simulink model "power_HEMS"  (R2017b)
settings: Solver=ode23tb  StartTime=0.0  StopTime=6  RelTol=1e-3  EnableMultiTasking=on
PreLoadFcn:
  | % Data of Solar Panel
  | %5000[W]/130[W]
  | % Total power generated by solar panel reaches 5[KW].
  | % each solar panel generates power 130[kW].
  | V = [0    40 80 120 160 180 200 217 240 260 280];
  | I = 5000/130*[0.68 0.675 0.67 0.665 0.660 0.655 0.640 0.6 0.48 0.28 0];
  | 
  | %subplot(211);plot(V,I);xlabel('Voltage[V]');ylabel('Current[a]')
  | %subplot(212);plot(V.*I);title('Power[W]')
  | 
  | % Sample Time[s]
  | Ts =5e-6;
  | 
  | 
  | %MPPT + PV Control
  | % PI control pamameter of Voltage control(Outer loop)
  | Kp_V = 50e-3;
  | Ki_V = 10;
  | 
  | % PI Control pamameter of Current control(Inner loop)
  | Kp_I = 25e-3;
  | Ki_I = 10;
  | 
  | % Utility Interconnection Control
  | % PI Control pamameter of Voltage control(Outer loop)
  | Kp_V2 = 0.01;
  | Ki_V2 = 25;
  | 
  | % PI control pamameter of Current control(Inner loop)
  | Kp_I2 = 0.01;
  | Ki_I2 = 25;
  | 
  | 
  | % Difference of voltege using in MPPT
  | dV = 0.5;
  | 
  | % Battery Control
  | % PI Control pamameter of Voltage control(Outer loop)
  | Kp_VB = 0.4;
  | Ki_VB = 2;
  | 
  | % PI control pamameter of Current control(Inner loop)
  | Kp_IB = 0.1;
  | Ki_IB = 0.5;
undefined symbols (not defined in the file or in its folder): Angle, Ion, Lithium, Magnitude, sigbuilder_block
libraries: powerlib x47, powerlib_meascontrol x8, simulink x6, electricdrivelib x1, simulink_extras x1
Description:
  | Copyright 2008-2017 The MathWorks, Inc.
settings Model: SimulationMode=accelerator  Creator=MathWorks  LastModifiedBy=solan
settings SolverCC: ZeroCrossControl=DisableAll  ZeroCrossAlgorithm=Adaptive
settings DataIOCC: LimitDataPoints=on  SaveFormat=Array  SignalLoggingSaveFormat=ModelDataLogs
settings OptimizationCC: ExpressionDepthLimit=2147483647  LifeSpan=inf
settings DebuggingCC: UnderspecifiedInitializationDetection=Classic  MergeDetectMultiDrivingBlocksExec=none  SolverPrmCheckMsg=warning  FcnCallInpInsideContextMsg=warning  AllowSymbolicDim=off  StateNameClashWarn=warning  SFUnexpectedBacktrackingDiag=warning  SFNoUnconditionalDefaultTransitionDiag=warning  SFExecutionAtInitializationDiag=none
settings HardwareCC: ProdBitPerPointer=32  ProdBitPerSizeT=32  ProdBitPerPtrDiffT=32  ProdLargestAtomicFloat=None  ProdIntDivRoundTo=Undefined  ProdEndianess=Unspecified  ProdWordSize=32  ProdHWDeviceType=32-bit Generic
settings ModelReferenceCC: PropagateSignalLabelsOutOfModel=off
settings SFSimCC: SimParseCustomCode=off
settings CodeAppCC: StateflowObjectComments=on
settings GRTTargetCC: TargetLangStandard=C89/C90 (ANSI)  GeneratePreprocessorConditionals=Disable all  CombineOutputUpdateFcns=off  GRTInterface=on
settings ConfigComp: CovMetricSettings=dw  CovHtmlReporting=on  CovSaveCumulativeToWorkspaceVar=on  CovSaveSingleToWorkspaceVar=on  CovShowResultsExplorer=off  CovExternalEMLEnable=off  CovSFcnEnable=off
settings SimscapeCC: SimscapeNormalizeSystem=off

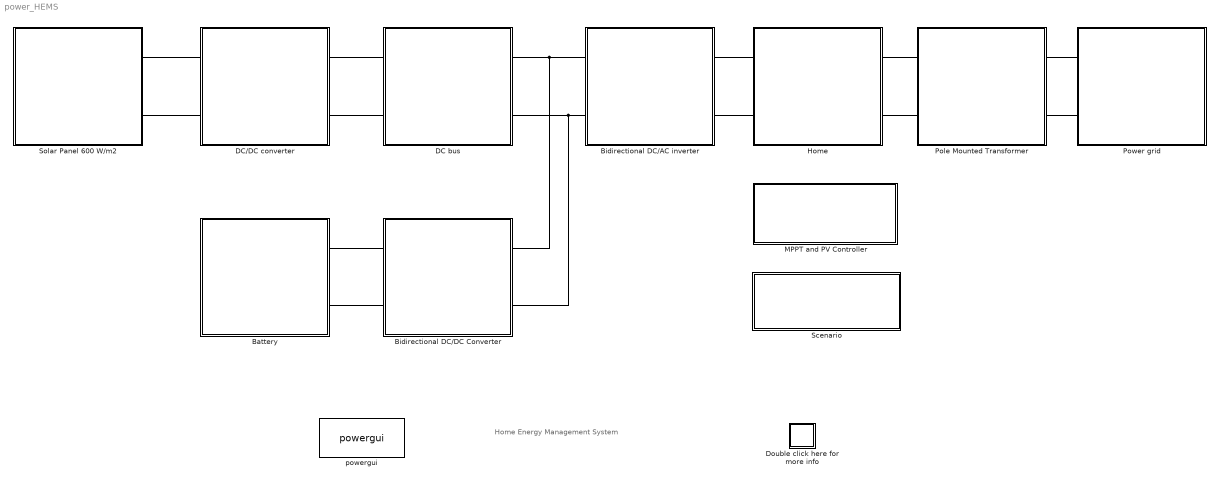
== system power_HEMS ==
  note: Home Energy Management System
  Battery : Subsystem
      mask Display: image(imread('Battery.jpg'))
  Bidirectional DC/AC inverter : Subsystem
      mask Display: image(imread('dcac.jpg'))
  Bidirectional DC/DC Converter : Subsystem
      mask Display: image(imread('bdcdc.jpg'))
  DC bus : Subsystem
      mask Display: image(imread('HVDC.jpg'))
  DC/DC converter : Subsystem
      mask Display: image(imread('dcdc.jpg'))
  Double click here for more info : Subsystem
      settings: OpenFcn=showdemo(bdroot(gcb))
      mask Display: disp('?')
  Home : Subsystem
      mask Display: image(imread('house.jpg'))
  MPPT and PV Controller : Subsystem
      mask Display: disp('Management system')
  Pole Mounted Transformer : Subsystem
      mask Display: image(imread('trans.jpg'))
  Power grid : Subsystem
      mask Display: image(imread('powersystem.jpg'))
  Scenario : Subsystem
      mask Display: disp('Additional\nScopes')
  Solar Panel 600 W/m2 : Subsystem
      mask Display: image(imread('pv.jpg'))
  powergui : powerlib/powergui  Priority=1  SimulationMode=Discrete  SampleTime=5e-6  frequency=60  Iterations=50  frequencyindice=0  Pbase=100e6  ErrMax=1e-4  UnitsV=kV  UnitsW=MW  buscounter=0  FunctionMessages=off  echomessages=off  EnableUseOfTLC=off  CurrentSourceSwitches=off  DisableSnubberDevices=off  DisableRonSwitches=off  DisableVfSwitches=off  DisplayEquations=off  SolverType=Tustin  Interpol=off  ExternalGateDelay=off  methode=off  Ts=0  x0status=blocks  SPID=off  SwTol=0  HookPort=off  RestoreLinks=warning  ResistiveCurrentMeasurement=off  Frange=[0:2:500]  Ylog=off  Xlog=on  ShowGrid=off  save=off  variable=ZData  structure=0  ZoomFFT=off  StartTime=0.0  cycles=1  DisplayStyle=1  fundamental=60  FreqAxis=off  MaxFrequency=1000  frequencyindicesteady=1  RmsSteady=1  display=off
  connections:
  DC/DC converter/RConn2 -- DC bus/LConn2
  Solar Panel 600 W/m2/RConn1 -- DC/DC converter/LConn1
  Bidirectional DC/AC inverter/RConn1 -- Home/LConn1
  Bidirectional DC/AC inverter/RConn2 -- Home/LConn2
  Bidirectional DC/DC Converter/RConn1 -- Battery/LConn1
  Bidirectional DC/DC Converter/RConn2 -- Battery/LConn2
  Power grid/LConn1 -- Pole Mounted Transformer/LConn1
  Home/RConn1 -- Pole Mounted Transformer/RConn1
  Home/RConn2 -- Pole Mounted Transformer/RConn2
  Power grid/LConn2 -- Pole Mounted Transformer/LConn2
  DC bus/RConn2 -- Bidirectional DC/AC inverter/LConn2 -- Bidirectional DC/DC Converter/LConn2
  Bidirectional DC/DC Converter/LConn1 -- DC bus/RConn1 -- Bidirectional DC/AC inverter/LConn1
  DC/DC converter/RConn1 -- DC bus/LConn1
  Solar Panel 600 W/m2/RConn2 -- DC/DC converter/LConn2

== system power_HEMS/Battery ==
  Battery : electricdrivelib/Extra Sources/Battery  BatType=Lithium-Ion  ShowTempParam=off  ThermalPreset=no  ShowAgeParam=off  NomV=200  NomQ=40  SOC=80  Batt_Tr=30/10  PresetModel=on  MaxQ=40  MinV=150  FullV=232.7974  Dis_rate=17.3913  R=0.05  Normal_OP=36.1739  expZone="[216.0772      1.965217]"  current=[1.5 3]  Units=Ampere-hour  Tci=20  NomT=25  T2=0  MaxQ2=2.208  FullV2=3.45  Normal_OP2=2.8  expZone2="[3.22        0.23]"  Rca=0.6  ti=1000  Dp=0  Neq0=0  Tsim=1e6  Ta1=25  Qeol=5.4*0.9  Reol=0.013333*1.2  Char_age=[2.3478, 3]  Dis_age=[2.3478, 10]  N1=1500  N2=10500  N3=1000  N4=1400  Ta2=45  N5=950
  Battery Status : Scope  NumInputPorts=4
  Bus Selector : BusSelector  OutputSignals=SOC (%),Current (A),Voltage (V)
  Product1 : Product  RndMeth=Zero
  + : PMIOPort  Port=1  Side=Left
  - : PMIOPort  Port=2  Side=Left
  tag scope: Power_Battery=global
  wires:
  Product1/1 -> [Power_Battery], Battery Status/4  "Power_Battery[W]"
  Bus Selector/1 -> Battery Status/1  "<SOC (%)>"
  Bus Selector/3 -> Product1/2, Battery Status/3  "<Voltage (V)>"
  Battery/1 -> Bus Selector/1
  Bus Selector/2 -> Product1/1, Battery Status/2  "<Current (A)>"
  connections:
  +/RConn1 -- Battery/LConn1
  -/RConn1 -- Battery/LConn2

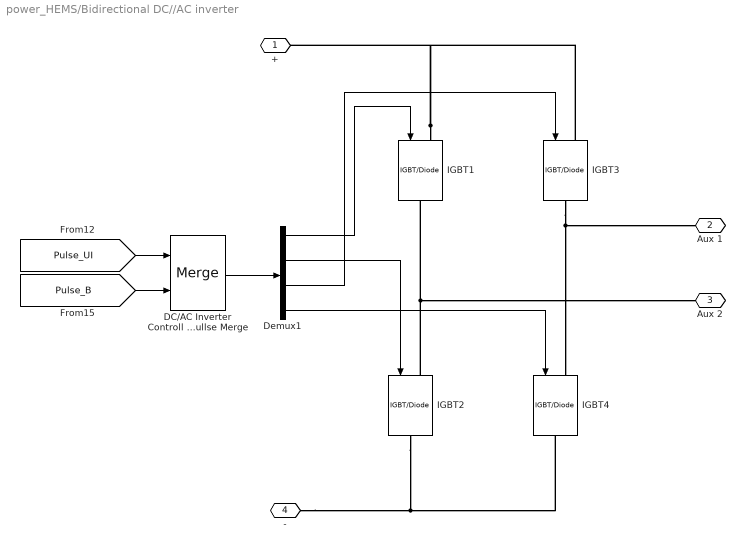
== system power_HEMS/Bidirectional DC//AC inverter ==
  DC/AC Inverter Controll Pullse Merge : Merge
  Demux1 : Demux
  IGBT{1..4} (4 alike) : powerlib/Power Electronics/IGBT//Diode  Ron=1e-3  Rs=1e5  Cs=inf  Measurements=off
  + : PMIOPort  Port=1  Side=Left
  Aux 1 : PMIOPort  Port=2  Side=Right
  Aux 2 : PMIOPort  Port=3  Side=Right
  - : PMIOPort  Port=4  Side=Left
  wires:
  Demux1/4 -> IGBT4/1
  Demux1/2 -> IGBT2/1
  Demux1/1 -> IGBT1/1
  [Pulse_B] -> DC/AC Inverter Controll Pullse Merge/2
  [Pulse_UI] -> DC/AC Inverter Controll Pullse Merge/1
  DC/AC Inverter Controll Pullse Merge/1 -> Demux1/1
  Demux1/3 -> IGBT3/1
  connections:
  IGBT2/RConn1 -- IGBT4/RConn1 -- -/RConn1
  IGBT3/RConn1 -- IGBT4/LConn1 -- Aux 1/RConn1
  IGBT2/LConn1 -- IGBT1/RConn1 -- Aux 2/RConn1
  IGBT1/LConn1 -- +/RConn1 -- IGBT3/LConn1

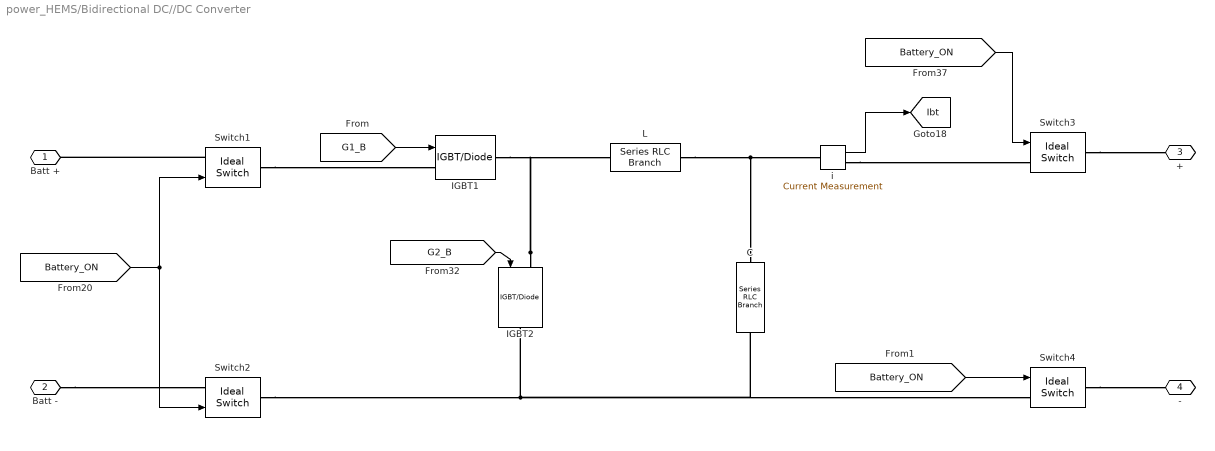
== system power_HEMS/Bidirectional DC//DC Converter ==
  C : powerlib/Elements/Series RLC Branch  LConnTagsString=__new0  RConnTagsString=__new0  BranchType=C  Resistance=1  Inductance=1e-3  SetiL0=off  InitialCurrent=0  Capacitance=1000e-6  Setx0=on  InitialVoltage=200  Measurements=None
  IGBT1 : powerlib/Power Electronics/IGBT//Diode  Ron=1e-3  Rs=1e5  Cs=inf  Measurements=off
  IGBT2 : powerlib/Power Electronics/IGBT//Diode  Ron=1e-3  Rs=1e5  Cs=inf  Measurements=off
  L : powerlib/Elements/Series RLC Branch  LConnTagsString=__new0  RConnTagsString=__new0  BranchType=L  Resistance=1  Inductance=470e-6*5  SetiL0=off  InitialCurrent=0  Capacitance=1000e-6  Setx0=off  InitialVoltage=0  Measurements=None
  Switch{1..4} (4 alike) : powerlib/Power Electronics/Ideal Switch  Ron=0.001  Lon=0  IC=0  Rs=1e6  Cs=inf  Measurements=off
  i : powerlib/Measurements/Current Measurement  PhasorSimulation=off  OutputType=Complex  PSBequivalent=0
  Batt + : PMIOPort  Port=1  Side=Left
  Batt - : PMIOPort  Port=2  Side=Left
  + : PMIOPort  Port=3  Side=Right
  - : PMIOPort  Port=4  Side=Right
  tag scope: Ibt=global
  wires:
  [G2_B] -> IGBT2/1
  [G1_B] -> IGBT1/1
  i/1 -> [Ibt]
  [Battery_ON] -> Switch3/1
  [Battery_ON] -> Switch1/1, Switch2/1
  [Battery_ON] -> Switch4/1
  connections:
  IGBT2/LConn1 -- L/RConn1 -- IGBT1/RConn1
  L/LConn1 -- i/LConn1 -- C/LConn1
  i/RConn1 -- Switch3/LConn1
  Switch3/RConn1 -- +/RConn1
  Switch4/RConn1 -- -/RConn1
  Switch1/RConn1 -- IGBT1/LConn1
  Switch4/LConn1 -- C/RConn1 -- IGBT2/RConn1 -- Switch2/RConn1
  Batt -/RConn1 -- Switch2/LConn1
  Switch1/LConn1 -- Batt +/RConn1

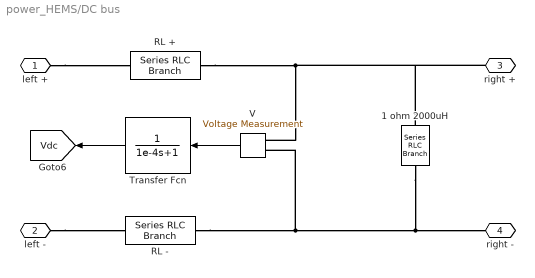
== system power_HEMS/DC bus ==
  1 ohm 2000uH : powerlib/Elements/Series RLC Branch  LConnTagsString=__new0  RConnTagsString=__new0  BranchType=RC  Resistance=1  Inductance=0  SetiL0=off  InitialCurrent=0  Capacitance=2000e-6  Setx0=on  InitialVoltage=370  Measurements=None
  RL + : powerlib/Elements/Series RLC Branch  LConnTagsString=__new0  RConnTagsString=__new0  BranchType=RL  Resistance=0.05  Inductance=470e-6  SetiL0=off  InitialCurrent=0  Capacitance=1e-6  Setx0=off  InitialVoltage=0  Measurements=None
  RL - : powerlib/Elements/Series RLC Branch  LConnTagsString=__new0  RConnTagsString=__new0  BranchType=RL  Resistance=0.05  Inductance=470e-6  SetiL0=off  InitialCurrent=0  Capacitance=1e-6  Setx0=off  InitialVoltage=0  Measurements=None
  Transfer Fcn : TransferFcn  Denominator=[1e-4 1]
  V : powerlib/Measurements/Voltage Measurement  PhasorSimulation=off  OutputType=Complex  PSBequivalent=0
  left + : PMIOPort  Port=1  Side=Left
  left - : PMIOPort  Port=2  Side=Left
  right + : PMIOPort  Port=3  Side=Right
  right - : PMIOPort  Port=4  Side=Right
  tag scope: Vdc=global
  wires:
  V/1 -> Transfer Fcn/1
  Transfer Fcn/1 -> [Vdc]
  connections:
  RL +/RConn1 -- 1 ohm 2000uH/LConn1 -- right +/RConn1 -- V/LConn1
  RL -/RConn1 -- 1 ohm 2000uH/RConn1 -- right -/RConn1 -- V/LConn2
  left +/RConn1 -- RL +/LConn1
  left -/RConn1 -- RL -/LConn1

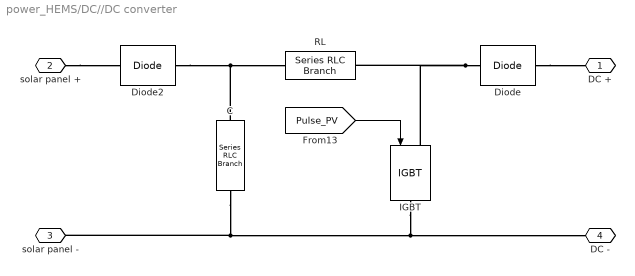
== system power_HEMS/DC//DC converter ==
  C : powerlib/Elements/Series RLC Branch  LConnTagsString=__new0  RConnTagsString=__new0  BranchType=C  Resistance=0.01  Inductance=1e-3  SetiL0=off  InitialCurrent=0  Capacitance=1000e-6  Setx0=on  InitialVoltage=200  Measurements=None
  Diode : powerlib/Power Electronics/Diode  Ron=0.001  Lon=0  Vf=1.1  IC=0  UseSnubber=off  Rs=500  Cs=250e-9  Measurements=off
  Diode2 : powerlib/Power Electronics/Diode  Ron=0.001  Lon=0  Vf=0.7  IC=0  UseSnubber=off  Rs=500  Cs=250e-9  Measurements=off
  IGBT : powerlib/Power Electronics/IGBT  Ron=0.001  Lon=0  Vf=1.1  Tf=1e-6  Tt=2e-6  IC=0  Rs=1e5  Cs=inf  Measurements=off
  RL : powerlib/Elements/Series RLC Branch  LConnTagsString=__new0  RConnTagsString=__new0  BranchType=RL  Resistance=0.05  Inductance=470e-6  SetiL0=off  InitialCurrent=0  Capacitance=1e-6  Setx0=off  InitialVoltage=0  Measurements=None
  DC + : PMIOPort  Port=1  Side=Right
  solar panel + : PMIOPort  Port=2  Side=Left
  solar panel - : PMIOPort  Port=3  Side=Left
  DC - : PMIOPort  Port=4  Side=Right
  wires:
  [Pulse_PV] -> IGBT/1
  connections:
  Diode/LConn1 -- RL/RConn1 -- IGBT/LConn1
  Diode/RConn1 -- DC +/RConn1
  Diode2/RConn1 -- C/LConn1 -- RL/LConn1
  solar panel +/RConn1 -- Diode2/LConn1
  C/RConn1 -- DC -/RConn1 -- IGBT/RConn1 -- solar panel -/RConn1

== system power_HEMS/Double click here for more info ==

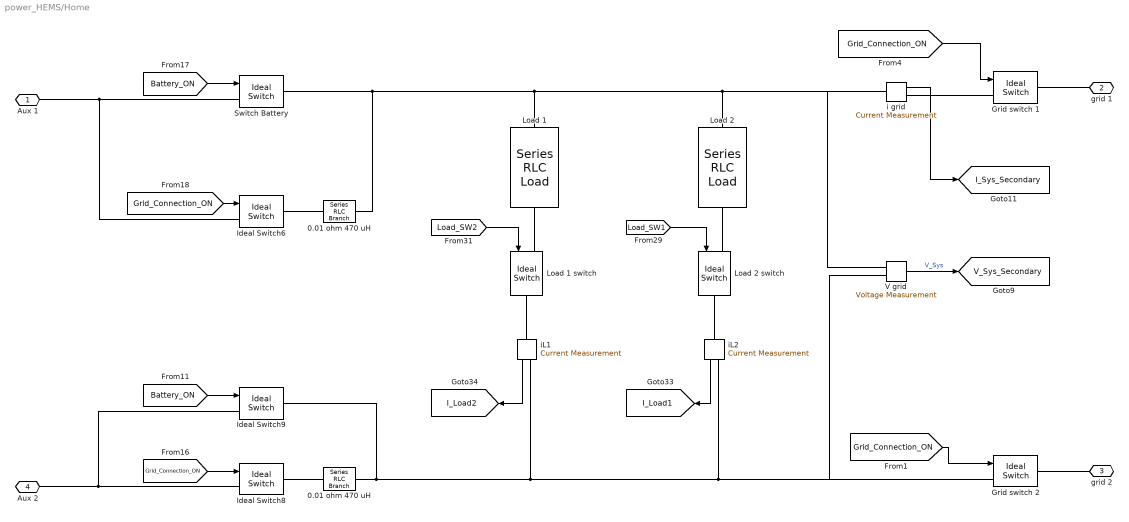
== system power_HEMS/Home ==
  0.01 ohm 470 uH : powerlib/Elements/Series RLC Branch  LConnTagsString=__new0  RConnTagsString=__new0  BranchType=RL  Resistance=0.01  Inductance=470e-06  SetiL0=off  InitialCurrent=0  Capacitance=[]  Setx0=off  InitialVoltage=0  Measurements=None
  "0.01 ohm 470 uH " : powerlib/Elements/Series RLC Branch  LConnTagsString=__new0  RConnTagsString=__new0  BranchType=RL  Resistance=0.01  Inductance=470e-06  SetiL0=off  InitialCurrent=0  Capacitance=[]  Setx0=off  InitialVoltage=0  Measurements=None
  Grid switch 1 : powerlib/Power Electronics/Ideal Switch  Ron=0.001  Lon=0  IC=0  Rs=1e5  Cs=inf  Measurements=off
  Grid switch 2 : powerlib/Power Electronics/Ideal Switch  Ron=0.001  Lon=0  IC=0  Rs=1e5  Cs=inf  Measurements=off
  Ideal Switch6 : powerlib/Power Electronics/Ideal Switch  Ron=0.001  Lon=0  IC=0  Rs=1e5  Cs=inf  Measurements=off
  Ideal Switch8 : powerlib/Power Electronics/Ideal Switch  Ron=0.001  Lon=0  IC=0  Rs=1e5  Cs=inf  Measurements=off
  Ideal Switch9 : powerlib/Power Electronics/Ideal Switch  Ron=0.001  Lon=0  IC=0  Rs=1e5  Cs=inf  Measurements=off
  Load 1 switch : powerlib/Power Electronics/Ideal Switch  Ron=0.001  Lon=0  IC=0  Rs=1e6  Cs=inf  Measurements=off
  "Load 1 " : powerlib/Elements/Series RLC Load  LConnTagsString=a  RConnTagsString=__new0  NominalVoltage=200  NominalFrequency=60  ActivePower=3e3  InductivePower=100  CapacitivePower=100  Setx0=off  InitialVoltage=0  SetiL0=off  InitialCurrent=0  Measurements=None  LoadType=constant Z
  Load 2 : powerlib/Elements/Series RLC Load  LConnTagsString=a  RConnTagsString=__new0  NominalVoltage=200  NominalFrequency=60  ActivePower=3e3  InductivePower=100  CapacitivePower=100  Setx0=off  InitialVoltage=0  SetiL0=off  InitialCurrent=0  Measurements=None  LoadType=constant Z
  Load 2 switch : powerlib/Power Electronics/Ideal Switch  Ron=0.001  Lon=0  IC=0  Rs=1e6  Cs=inf  Measurements=off
  Switch Battery : powerlib/Power Electronics/Ideal Switch  Ron=0.001  Lon=0  IC=0  Rs=1e5  Cs=inf  Measurements=off
  V grid : powerlib/Measurements/Voltage Measurement  PhasorSimulation=off  OutputType=Complex  PSBequivalent=0
  i grid : powerlib/Measurements/Current Measurement  PhasorSimulation=off  OutputType=Complex  PSBequivalent=0
  iL1 : powerlib/Measurements/Current Measurement  PhasorSimulation=off  OutputType=Complex  PSBequivalent=0
  iL2 : powerlib/Measurements/Current Measurement  PhasorSimulation=off  OutputType=Complex  PSBequivalent=0
  Aux 1 : PMIOPort  Port=1  Side=Left
  grid 1 : PMIOPort  Port=2  Side=Right
  grid 2 : PMIOPort  Port=3  Side=Right
  Aux 2 : PMIOPort  Port=4  Side=Left
  tag scope: I_Load1=global, I_Load2=global, I_Sys_Secondary=global, V_Sys_Secondary=global
  wires:
  i grid/1 -> [I_Sys_Secondary]
  [Load_SW1] -> Load 2 switch/1
  V grid/1 -> [V_Sys_Secondary]  "V_Sys"
  [Load_SW2] -> Load 1 switch/1
  iL2/1 -> [I_Load1]
  iL1/1 -> [I_Load2]
  [Grid_Connection_ON] -> Grid switch 1/1
  [Battery_ON] -> Ideal Switch9/1
  [Grid_Connection_ON] -> Ideal Switch8/1
  [Grid_Connection_ON] -> Ideal Switch6/1
  [Battery_ON] -> Switch Battery/1
  [Grid_Connection_ON] -> Grid switch 2/1
  connections:
  Load 2/LConn1 -- Load 2 switch/LConn1
  "Load 1 "/LConn1 -- Load 1 switch/LConn1
  iL1/LConn1 -- Load 1 switch/RConn1
  iL2/LConn1 -- Load 2 switch/RConn1
  Grid switch 1/RConn1 -- grid 1/RConn1
  i grid/RConn1 -- Grid switch 1/LConn1
  Grid switch 2/RConn1 -- grid 2/RConn1
  0.01 ohm 470 uH/RConn1 -- "Load 1 "/RConn1 -- V grid/LConn1 -- i grid/LConn1 -- Load 2/RConn1 -- Switch Battery/RConn1
  "0.01 ohm 470 uH "/RConn1 -- Grid switch 2/LConn1 -- V grid/LConn2 -- iL2/RConn1 -- iL1/RConn1 -- Ideal Switch9/RConn1
  Ideal Switch6/RConn1 -- 0.01 ohm 470 uH/LConn1
  Ideal Switch8/RConn1 -- "0.01 ohm 470 uH "/LConn1
  Ideal Switch9/LConn1 -- Aux 2/RConn1 -- Ideal Switch8/LConn1
  Aux 1/RConn1 -- Ideal Switch6/LConn1 -- Switch Battery/LConn1

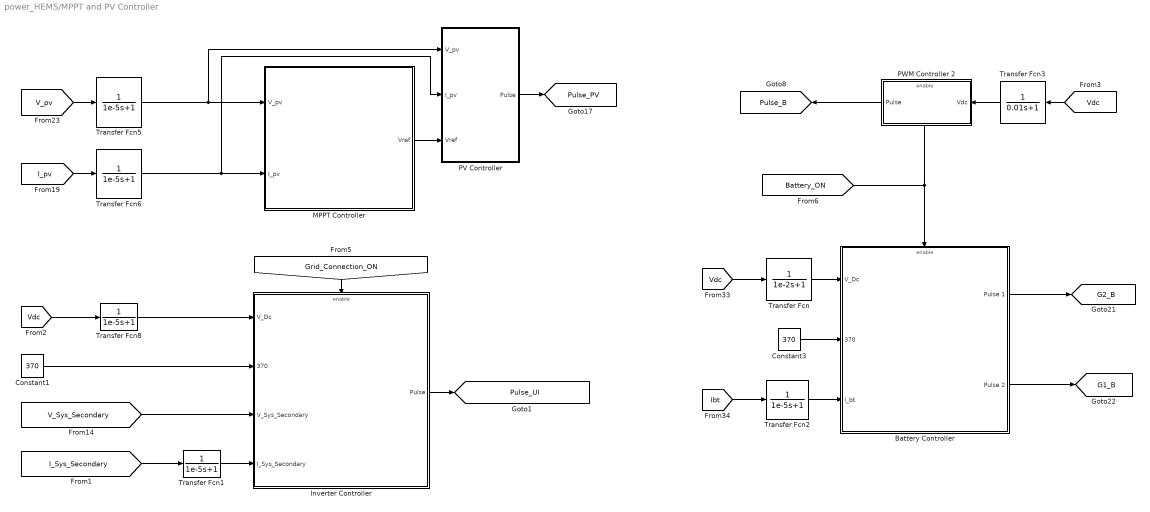
== system power_HEMS/MPPT and PV Controller ==
  Battery Controller : Subsystem
  Constant1 : Constant  Value=370
  Constant3 : Constant  Value=370
  Inverter Controller : Subsystem
  MPPT Controller : Stateflow chart  TreatAsAtomicUnit=on
  PV Controller : Subsystem
  PWM Controller 2 : Subsystem
  Transfer Fcn : TransferFcn  Denominator=[1e-2 1]
  Transfer Fcn{1..2,5..6,8} (5 alike) : TransferFcn  Denominator=[1e-5 1]
  Transfer Fcn3 : TransferFcn  Denominator=[0.01 1]
  tag scope: G1_B=global, G2_B=global, Pulse_B=global, Pulse_PV=global, Pulse_UI=global
  wires:
  MPPT Controller/1(Vref) -> PV Controller/3(Vref)
  [V_pv] -> Transfer Fcn5/1
  [I_pv] -> Transfer Fcn6/1
  PV Controller/1(Pulse) -> [Pulse_PV]
  Transfer Fcn5/1 -> MPPT Controller/1(V_pv), PV Controller/1(V_pv)
  Transfer Fcn6/1 -> MPPT Controller/2(I_pv), PV Controller/2(I_pv)
  [Vdc] -> Transfer Fcn8/1
  [Grid_Connection_ON] -> Inverter Controller/Enable
  [I_Sys_Secondary] -> Transfer Fcn1/1
  Transfer Fcn1/1 -> Inverter Controller/4(I_Sys_Secondary)
  [V_Sys_Secondary] -> Inverter Controller/3(V_Sys_Secondary)
  Inverter Controller/1(Pulse) -> [Pulse_UI]
  Constant1/1 -> Inverter Controller/2(370)
  Transfer Fcn8/1 -> Inverter Controller/1(V_Dc)
  Constant3/1 -> Battery Controller/2(370)
  PWM Controller 2/1(Pulse) -> [Pulse_B]
  [Vdc] -> Transfer Fcn3/1
  [Battery_ON] -> Battery Controller/Enable, PWM Controller 2/Enable
  [Ibt] -> Transfer Fcn2/1
  [Vdc] -> Transfer Fcn/1
  Transfer Fcn3/1 -> PWM Controller 2/1(Vdc)
  Transfer Fcn2/1 -> Battery Controller/3(I_bt)
  Transfer Fcn/1 -> Battery Controller/1(V_Dc)
  Battery Controller/2(Pulse 2) -> [G1_B]
  Battery Controller/1(Pulse 1) -> [G2_B]

== system power_HEMS/Pole Mounted Transformer ==
  note: HOUSE
  note: GRID
  Multi-Winding Transformer : powerlib/Elements/Multi-Winding Transformer  LeftWindings=1  RightWindings=2  TappedWindings=no taps  NumberOfTaps=2  SetSaturation=off  Hysteresis=off  DataFile='hysteresis.mat'  Measurements=None  UNITS=pu  NominalPower=[75e3 60]  NominalVoltages=[ 6600 100 100 ]  WindingResistances="[ 0.00005  0.00005  0.00005  0.00005]"  WindingInductances="[ 0.0002  0.0002  0.0002  0.0002 ]  * 100 % to eliminate the Matrix is close to similar  warning"  Rm=50  Lm=50  Saturation=[ 0,0 ; 0.0024,1.2 ; 1.0,1.52 ]  MoreParameters=off  BreakLoop=off  DataType=off  InitialFlux=0  TransfoNumber=1
      settings: SourceProductName=Simscape Power Systems  SourceProductBaseCode=PS
  Conn1 : PMIOPort  Port=1  Side=Left
  Conn2 : PMIOPort  Port=2  Side=Right
  Conn3 : PMIOPort  Port=3  Side=Right
  Conn4 : PMIOPort  Port=4  Side=Left
  connections:
  Conn2/RConn1 -- Multi-Winding Transformer/RConn1
  Conn3/RConn1 -- Multi-Winding Transformer/RConn4
  Conn1/RConn1 -- Multi-Winding Transformer/LConn1
  Conn4/RConn1 -- Multi-Winding Transformer/LConn2
  Multi-Winding Transformer/RConn2 -- Multi-Winding Transformer/RConn3

== system power_HEMS/Power grid ==
  6.6kv Transformer : powerlib/Elements/Three-Phase Transformer (Two Windings)  Winding1Connection=Yg  Winding2Connection=Y  CoreType=Three single-phase transformers  SetSaturation=off  Hysteresis=off  DataFile='hysteresis'  SetInitialFlux=off  Measurements=None  UNITS=pu  NominalPower=[ 10e6 , 60 ]  Winding1=[ 66e3 , 0.002 , 0.08 ]  Winding2=[6.6e3 , 0.002 , 0.08 ]  Rm=500  Lm=500  L0=0.5  Saturation=[ 0,0 ; 0.0024,1.2 ; 1.0,1.52 ]  InitialFluxes=[ 0.8 , -0.8 , 0.7 ]  MoreParameters=off  BreakLoop=on  DataType=off  TransfoNumber=1
  66 kV : powerlib/Electrical Sources/Three-Phase Source  InternalConnection=Yg  VoltagePhases=off  Voltage=66e3  PhaseAngle=0  Voltage_phases=[25e3 25e3 25e3]/sqrt(3)  PhaseAngles_phases=[0 -120 +120]  Frequency=60  NonIdealSource=on  SpecifyImpedance=on  Resistance=0.8929  Inductance=16.58e-3  ShortCircuitLevel=100e6  BaseVoltage=25e3  XRratio=7  BusType=swing  Pref=0  Qref=0  Prefabc=[10e3, 10e3, 10e3]  Qrefabc=[0, 0, 0]  Qmin=-inf  Qmax=inf
  SEND : powerlib/Elements/Three-Phase PI Section Line  LConnTagsString=a|b|c  RConnTagsString=A|B|C  Frequency=60  Resistances=[ 0.01273 0.3864]  Inductances="[ 0.9337e-3  4.1264e-3]"  Capacitances=[12.74e-9 7.751e-9]  Length=1
      settings: SourceProductName=Simscape Power Systems
  ia : powerlib/Measurements/Current Measurement  PhasorSimulation=off  OutputType=Magnitude-Angle  PSBequivalent=0
  vab : powerlib/Measurements/Voltage Measurement  PhasorSimulation=off  OutputType=Magnitude-Angle  PSBequivalent=0
  Conn1 : PMIOPort  Port=1  Side=Left
  Conn2 : PMIOPort  Port=2  Side=Left
  tag scope: I_Sys_Primary=global, V_Sys_Primary=global
  wires:
  ia/1 -> [I_Sys_Primary]
  vab/1 -> [V_Sys_Primary]
  connections:
  6.6kv Transformer/RConn2 -- SEND/LConn2
  6.6kv Transformer/RConn3 -- SEND/LConn3
  6.6kv Transformer/RConn1 -- SEND/LConn1
  66 kV/RConn2 -- 6.6kv Transformer/LConn2
  66 kV/RConn1 -- 6.6kv Transformer/LConn1
  66 kV/RConn3 -- 6.6kv Transformer/LConn3
  SEND/RConn3 -- Conn2/RConn1 -- vab/LConn2
  ia/LConn1 -- SEND/RConn1
  vab/LConn1 -- Conn1/RConn1 -- ia/RConn1

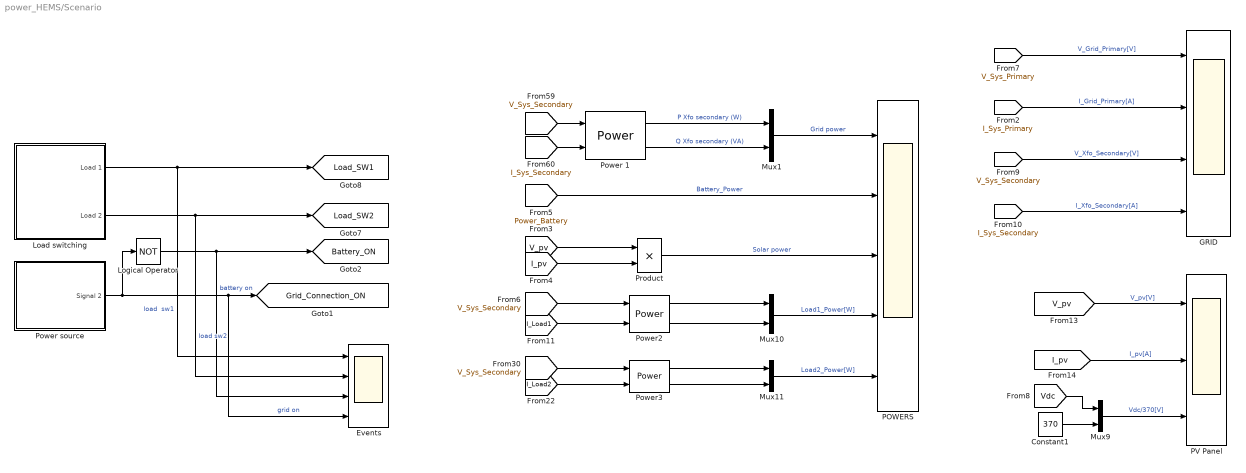
== system power_HEMS/Scenario ==
  Constant1 : Constant  Value=370
  Events : Scope  NumInputPorts=4
  GRID : Scope  NumInputPorts=4
  Load switching : Subsystem  Tag=STV Subsys  LoadFcn=sigbuilder_block('load');  StartFcn=sigbuilder_block('start');  StopFcn=sigbuilder_block('stop');  ClipboardFcn=sigbuilder_block('clipboard');  mask(Sigbuilder block){tuvar=[0:10]}
      mask help: Simulink:masks:SigbuilderBlock_MD
      mask init:
      | if ~strcmp(get_param(bdroot(gcbh),'SimulationStatus'),'stopped') tuvar = sigbuilder_block('maskInit'); end
      settings: CopyFcn=sigbuilder_block('copy');  DeleteFcn=sigbuilder_block('delete');  ModelCloseFcn=sigbuilder_block('modelClose');  PreSaveFcn=sigbuilder_block('preSave');  PauseFcn=sigbuilder_block('pause');  ContinueFcn=sigbuilder_block('continue');  NameChangeFcn=sigbuilder_block('namechange');  OpenFcn=sigbuilder_block('open',[57 105.75 1180.5 663.75 ]);  CloseFcn=sigbuilder_block('close');
      mask Display: plot(0, 0, 100, 100,[2, 2, 32, 32, 2], [68, 8, 8, 68, 68],[32, 2], [38, 38], [32, 19, 2],[53, 60, 44], [32, 17, 17, 2],[16, 16, 31, 31]);txt = getActiveGroup(gcbh);text(2, 100, txt,'verticalAlignment', 'top');
  Logical Operator : Logic  Operator=NOT  AllPortsSameDT=off  OutDataTypeStr=boolean
  Mux{1,9..11} (4 alike) : Mux  Inputs=2
  POWERS : Scope  NumInputPorts=5
  PV Panel : Scope  NumInputPorts=3
  Power 1 : powerlib_meascontrol/Measurements/Power  Freq=60  Vinit=[1, 0]  Iinit=[1, 0]  Ts=0
      settings: SourceProductName=Simscape Power Systems
  Power source : Subsystem  Tag=STV Subsys  LoadFcn=sigbuilder_block('load');  StartFcn=sigbuilder_block('start');  StopFcn=sigbuilder_block('stop');  ClipboardFcn=sigbuilder_block('clipboard');  mask(Sigbuilder block){tuvar=[0:10]}
      mask help: Simulink:masks:SigbuilderBlock_MD
      mask init:
      | if ~strcmp(get_param(bdroot(gcbh),'SimulationStatus'),'stopped') tuvar = sigbuilder_block('maskInit'); end
      settings: CopyFcn=sigbuilder_block('copy');  DeleteFcn=sigbuilder_block('delete');  ModelCloseFcn=sigbuilder_block('modelClose');  PreSaveFcn=sigbuilder_block('preSave');  PauseFcn=sigbuilder_block('pause');  ContinueFcn=sigbuilder_block('continue');  NameChangeFcn=sigbuilder_block('namechange');  OpenFcn=sigbuilder_block('open',[436.966 199.241 549.931 400.345 ]);  CloseFcn=sigbuilder_block('close');
      mask Display: plot(0, 0, 100, 100,[2, 2, 32, 32, 2], [68, 8, 8, 68, 68],[32, 2], [38, 38], [32, 19, 2],[53, 60, 44], [32, 17, 17, 2],[16, 16, 31, 31]);txt = getActiveGroup(gcbh);text(2, 100, txt,'verticalAlignment', 'top');
  Power2 : powerlib_meascontrol/Measurements/Power  Freq=60  Vinit=[1, 0]  Iinit=[1, 0]  Ts=0
      settings: SourceProductName=Simscape Power Systems
  Power3 : powerlib_meascontrol/Measurements/Power  Freq=60  Vinit=[1, 0]  Iinit=[1, 0]  Ts=0
      settings: SourceProductName=Simscape Power Systems
  Product : Product  RndMeth=Zero
  tag scope: Battery_ON=global, Grid_Connection_ON=global, Load_SW1=global, Load_SW2=global
  wires:
  Load switching/2(Load 2) -> [Load_SW2], Events/2  "load sw2"
  Logical Operator/1 -> Events/3, [Battery_ON]  "battery on"
  Power source/1(Signal 2) -> Events/4, [Grid_Connection_ON], Logical Operator/1  "grid on"
  Load switching/1(Load 1) -> [Load_SW1], Events/1  "load  sw1"
  [Vdc] -> Mux9/1
  Constant1/1 -> Mux9/2
  Mux9/1 -> PV Panel/3  "Vdc/370[V]"
  [V_Sys_Primary] -> GRID/1  "V_Grid_Primary[V]"
  [I_Sys_Primary] -> GRID/2  "I_Grid_Primary[A]"
  [V_Sys_Secondary] -> GRID/3  "V_Xfo_Secondary[V]"
  [I_Sys_Secondary] -> GRID/4  "I_Xfo_Secondary[A]"
  [V_pv] -> PV Panel/1  "V_pv[V]"
  [I_pv] -> PV Panel/2  "I_pv[A]"
  [V_pv] -> Product/1
  [I_pv] -> Product/2
  Product/1 -> POWERS/3  "Solar power"
  [Power_Battery] -> POWERS/2  "Battery_Power"
  [V_Sys_Secondary] -> Power 1/1
  [I_Sys_Secondary] -> Power 1/2
  [V_Sys_Secondary] -> Power2/1
  [I_Load1] -> Power2/2
  Mux10/1 -> POWERS/4  "Load1_Power[W]"
  [V_Sys_Secondary] -> Power3/1
  [I_Load2] -> Power3/2
  Mux11/1 -> POWERS/5  "Load2_Power[W]"
  Power2/1 -> Mux10/1
  Power2/2 -> Mux10/2
  Power3/1 -> Mux11/1
  Power3/2 -> Mux11/2
  Mux1/1 -> POWERS/1  "Grid power"
  Power 1/1 -> Mux1/1  "P Xfo secondary (W)"
  Power 1/2 -> Mux1/2  "Q Xfo secondary (VA)"

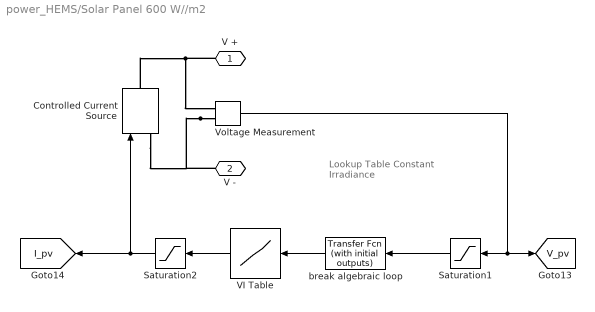
== system power_HEMS/Solar Panel 600 W//m2 ==
  note: Lookup Table
      | Constant Irradiance
  Controlled Current Source : powerlib/Electrical Sources/Controlled Current Source  Initialize=on  Source_Type=DC  Amplitude=0  Phase=0  Frequency=0  Measurements=None
  Saturation1 : Saturate  UpperLimit=100  LowerLimit=10
  Saturation2 : Saturate  UpperLimit=100  LowerLimit=10
  VI Table : Lookup  InputValues=V  Table=I
  Voltage Measurement : powerlib/Measurements/Voltage Measurement  PhasorSimulation=off  OutputType=Complex  PSBequivalent=0
  break algebraic loop : simulink_extras/Additional Linear/Transfer Fcn (with initial outputs)  N=[1]  D="[1e-6  1]"  Y0=0  U0=0
  V + : PMIOPort  Port=1  Side=Right
  V - : PMIOPort  Port=2  Side=Right
  tag scope: I_pv=global, V_pv=global
  wires:
  break algebraic loop/1 -> VI Table/1
  VI Table/1 -> Saturation2/1
  Saturation1/1 -> break algebraic loop/1
  Saturation2/1 -> Controlled Current Source/1, [I_pv]
  Voltage Measurement/1 -> Saturation1/1, [V_pv]
  connections:
  Voltage Measurement/LConn2 -- V -/RConn1 -- Controlled Current Source/LConn1
  Controlled Current Source/RConn1 -- Voltage Measurement/LConn1 -- V +/RConn1

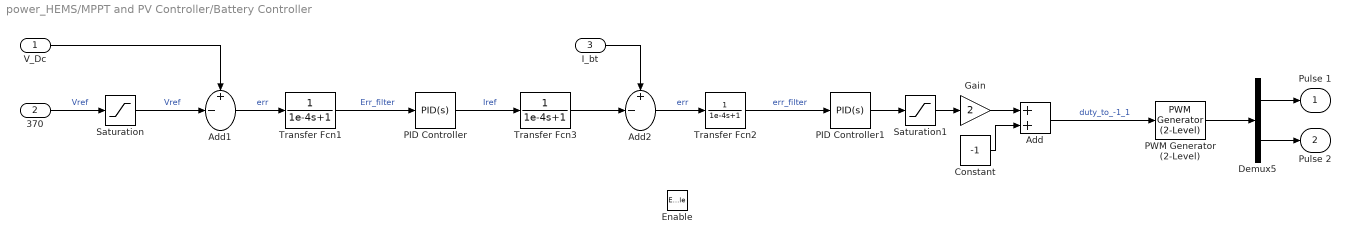
== system power_HEMS/MPPT and PV Controller/Battery Controller ==
  V_Dc : Inport
  370 : Inport  Port=2
  I_bt : Inport  Port=3
  Enable : EnablePort  StatesWhenEnabling=reset
  Add : Sum
  Add1 : Sum  Inputs=+-|
  Add2 : Sum  Inputs=+-|
  Constant : Constant  Value=-1
  Demux5 : Demux  Outputs=2
  Gain : Gain  Gain=2
  PID Controller : simulink/Continuous/PID Controller  Controller=PID  TimeDomain=Continuous-time  SampleTime=-1  IntegratorMethod=Forward Euler  FilterMethod=Forward Euler  Form=Parallel  UseFilter=on  ControllerParametersSource=internal  P=Kp_VB  I=Ki_VB  D=0  N=100  InitialConditionSource=internal  InitialConditionForIntegrator=0  InitialConditionForFilter=0  ExternalReset=none  LimitOutput=off  UpperSaturationLimit=inf  LowerSaturationLimit=-inf  LinearizeAsGain=off  AntiWindupMode=none  Kb=1  TrackingMode=off  Kt=1  PParamMin=[]  PParamMax=[]  IParamMin=[]  IParamMax=[]  DParamMin=[]  DParamMax=[]  NParamMin=[]  NParamMax=[]  KbParamMin=[]  KbParamMax=[]  KtParamMin=[]  KtParamMax=[]  POutMin=[]  POutMax=[]  IOutMin=[]  IOutMax=[]  DOutMin=[]  DOutMax=[]  NOutMin=[]  NOutMax=[]  KbOutMin=[]  KbOutMax=[]  KtOutMin=[]  KtOutMax=[]  IntegratorOutMin=[]  IntegratorOutMax=[]  FilterOutMin=[]  FilterOutMax=[]  SumOutMin=[]  SumOutMax=[]  SumI1OutMin=[]  SumI1OutMax=[]  SumI2OutMin=[]  SumI2OutMax=[]  SumI3OutMin=[]  SumI3OutMax=[]  SumDOutMin=[]  SumDOutMax=[]  SaturationOutMin=[]  SaturationOutMax=[]  IntegratorContinuousStateAttributes=''  IntegratorStateMustResolveToSignalObject=off  IntegratorRTWStateStorageClass=Auto  FilterContinuousStateAttributes=''  FilterStateMustResolveToSignalObject=off  FilterRTWStateStorageClass=Auto  DifferentiatorICPrevScaledInput=0  DifferentiatorOutMin=[]  DifferentiatorOutMax=[]  InitialConditionSetting=State (most efficient)  FilterDiffOutCoefMin=[]  FilterDiffOutCoefMax=[]  SumDenOutMin=[]  SumDenOutMax=[]  SumNumOutMin=[]  SumNumOutMax=[]  ReciprocalOutMin=[]  ReciprocalOutMax=[]  DivideOutMin=[]  DivideOutMax=[]  TunerSelectOption=Transfer Function Based (PID Tuner App)
  PID Controller1 : simulink/Continuous/PID Controller  Controller=PID  TimeDomain=Continuous-time  SampleTime=-1  IntegratorMethod=Forward Euler  FilterMethod=Forward Euler  Form=Parallel  UseFilter=on  ControllerParametersSource=internal  P=Kp_IB  I=Ki_IB  D=0  N=100  InitialConditionSource=internal  InitialConditionForIntegrator=0  InitialConditionForFilter=0  ExternalReset=none  LimitOutput=off  UpperSaturationLimit=inf  LowerSaturationLimit=-inf  LinearizeAsGain=off  AntiWindupMode=none  Kb=1  TrackingMode=off  Kt=1  PParamMin=[]  PParamMax=[]  IParamMin=[]  IParamMax=[]  DParamMin=[]  DParamMax=[]  NParamMin=[]  NParamMax=[]  KbParamMin=[]  KbParamMax=[]  KtParamMin=[]  KtParamMax=[]  POutMin=[]  POutMax=[]  IOutMin=[]  IOutMax=[]  DOutMin=[]  DOutMax=[]  NOutMin=[]  NOutMax=[]  KbOutMin=[]  KbOutMax=[]  KtOutMin=[]  KtOutMax=[]  IntegratorOutMin=[]  IntegratorOutMax=[]  FilterOutMin=[]  FilterOutMax=[]  SumOutMin=[]  SumOutMax=[]  SumI1OutMin=[]  SumI1OutMax=[]  SumI2OutMin=[]  SumI2OutMax=[]  SumI3OutMin=[]  SumI3OutMax=[]  SumDOutMin=[]  SumDOutMax=[]  SaturationOutMin=[]  SaturationOutMax=[]  IntegratorContinuousStateAttributes=''  IntegratorStateMustResolveToSignalObject=off  IntegratorRTWStateStorageClass=Auto  FilterContinuousStateAttributes=''  FilterStateMustResolveToSignalObject=off  FilterRTWStateStorageClass=Auto  DifferentiatorICPrevScaledInput=0  DifferentiatorOutMin=[]  DifferentiatorOutMax=[]  InitialConditionSetting=State (most efficient)  FilterDiffOutCoefMin=[]  FilterDiffOutCoefMax=[]  SumDenOutMin=[]  SumDenOutMax=[]  SumNumOutMin=[]  SumNumOutMax=[]  ReciprocalOutMin=[]  ReciprocalOutMax=[]  DivideOutMin=[]  DivideOutMax=[]  TunerSelectOption=Transfer Function Based (PID Tuner App)
  PWM Generator (2-Level) : powerlib_meascontrol/Pulse & Signal Generators/PWM Generator (2-Level)  ModulatorType=Single-phase half-bridge (2 pulses)  ModulatorMode=Unsynchronized  Fc=10000  Pc=90  nF=27  MinMax="[ -1  1 ]"  SamplingTechnique=Natural  ModulatingSignals=off  m=0.8  Freq=60  Phase=0  Ts=0  ShowCarrierOutport=off
      settings: SourceProductName=Simscape Power Systems
  Saturation : Saturate  UpperLimit=370  LowerLimit=0
  Saturation1 : Saturate  UpperLimit=1  LowerLimit=0
  Transfer Fcn1 : TransferFcn  Denominator=[1e-4 1]
  Transfer Fcn2 : TransferFcn  Denominator=[1e-4 1]
  Transfer Fcn3 : TransferFcn  Denominator=[1e-4 1]
  Pulse 1 : Outport  OutputWhenDisabled=reset  InitialOutput=0
  Pulse 2 : Outport  Port=2  OutputWhenDisabled=reset  InitialOutput=0
  wires:
  370/1 -> Saturation/1  "Vref"
  Add/1 -> PWM Generator (2-Level)/1  "duty_to_-1_1"
  Gain/1 -> Add/1
  Constant/1 -> Add/2
  Saturation/1 -> Add1/2  "Vref"
  V_Dc/1 -> Add1/1
  Add1/1 -> Transfer Fcn1/1  "err"
  I_bt/1 -> Add2/1
  Add2/1 -> Transfer Fcn2/1  "err"
  PID Controller1/1 -> Saturation1/1
  Transfer Fcn1/1 -> PID Controller/1  "Err_filter"
  Transfer Fcn2/1 -> PID Controller1/1  "err_filter"
  PID Controller/1 -> Transfer Fcn3/1  "Iref"
  Transfer Fcn3/1 -> Add2/2
  Saturation1/1 -> Gain/1
  Demux5/1 -> Pulse 1/1
  Demux5/2 -> Pulse 2/1
  PWM Generator (2-Level)/1 -> Demux5/1

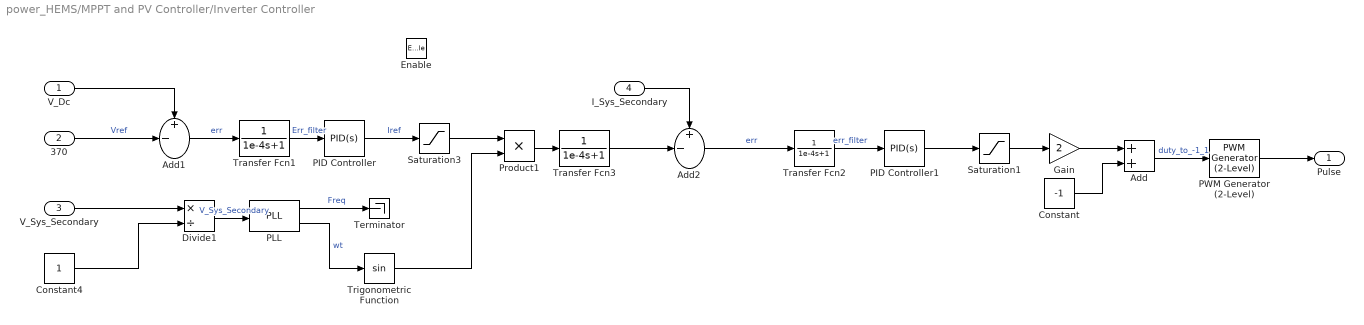
== system power_HEMS/MPPT and PV Controller/Inverter Controller ==
  V_Dc : Inport
  370 : Inport  Port=2
  V_Sys_Secondary : Inport  Port=3
  I_Sys_Secondary : Inport  Port=4
  Enable : EnablePort  StatesWhenEnabling=reset
  Add : Sum
  Add1 : Sum  Inputs=+-|
  Add2 : Sum  Inputs=+-|
  Constant : Constant  Value=-1
  Constant4 : Constant
  Divide1 : Product  Inputs=*/
  Gain : Gain  Gain=2
  PID Controller : simulink/Continuous/PID Controller  Controller=PID  TimeDomain=Continuous-time  SampleTime=-1  IntegratorMethod=Forward Euler  FilterMethod=Forward Euler  Form=Parallel  UseFilter=on  ControllerParametersSource=internal  P=Kp_V2*10  I=Ki_V2*10  D=0  N=100  InitialConditionSource=internal  InitialConditionForIntegrator=0  InitialConditionForFilter=0  ExternalReset=none  LimitOutput=off  UpperSaturationLimit=inf  LowerSaturationLimit=-inf  LinearizeAsGain=off  AntiWindupMode=none  Kb=1  TrackingMode=off  Kt=1  PParamMin=[]  PParamMax=[]  IParamMin=[]  IParamMax=[]  DParamMin=[]  DParamMax=[]  NParamMin=[]  NParamMax=[]  KbParamMin=[]  KbParamMax=[]  KtParamMin=[]  KtParamMax=[]  POutMin=[]  POutMax=[]  IOutMin=[]  IOutMax=[]  DOutMin=[]  DOutMax=[]  NOutMin=[]  NOutMax=[]  KbOutMin=[]  KbOutMax=[]  KtOutMin=[]  KtOutMax=[]  IntegratorOutMin=[]  IntegratorOutMax=[]  FilterOutMin=[]  FilterOutMax=[]  SumOutMin=[]  SumOutMax=[]  SumI1OutMin=[]  SumI1OutMax=[]  SumI2OutMin=[]  SumI2OutMax=[]  SumI3OutMin=[]  SumI3OutMax=[]  SumDOutMin=[]  SumDOutMax=[]  SaturationOutMin=[]  SaturationOutMax=[]  IntegratorContinuousStateAttributes=''  IntegratorStateMustResolveToSignalObject=off  IntegratorRTWStateStorageClass=Auto  FilterContinuousStateAttributes=''  FilterStateMustResolveToSignalObject=off  FilterRTWStateStorageClass=Auto  DifferentiatorICPrevScaledInput=0  DifferentiatorOutMin=[]  DifferentiatorOutMax=[]  InitialConditionSetting=State (most efficient)  FilterDiffOutCoefMin=[]  FilterDiffOutCoefMax=[]  SumDenOutMin=[]  SumDenOutMax=[]  SumNumOutMin=[]  SumNumOutMax=[]  ReciprocalOutMin=[]  ReciprocalOutMax=[]  DivideOutMin=[]  DivideOutMax=[]  TunerSelectOption=Transfer Function Based (PID Tuner App)
  PID Controller1 : simulink/Continuous/PID Controller  Controller=PID  TimeDomain=Continuous-time  SampleTime=-1  IntegratorMethod=Forward Euler  FilterMethod=Forward Euler  Form=Parallel  UseFilter=on  ControllerParametersSource=internal  P=Kp_I2  I=Ki_I2  D=0  N=100  InitialConditionSource=internal  InitialConditionForIntegrator=0  InitialConditionForFilter=0  ExternalReset=none  LimitOutput=off  UpperSaturationLimit=inf  LowerSaturationLimit=-inf  LinearizeAsGain=off  AntiWindupMode=none  Kb=1  TrackingMode=off  Kt=1  PParamMin=[]  PParamMax=[]  IParamMin=[]  IParamMax=[]  DParamMin=[]  DParamMax=[]  NParamMin=[]  NParamMax=[]  KbParamMin=[]  KbParamMax=[]  KtParamMin=[]  KtParamMax=[]  POutMin=[]  POutMax=[]  IOutMin=[]  IOutMax=[]  DOutMin=[]  DOutMax=[]  NOutMin=[]  NOutMax=[]  KbOutMin=[]  KbOutMax=[]  KtOutMin=[]  KtOutMax=[]  IntegratorOutMin=[]  IntegratorOutMax=[]  FilterOutMin=[]  FilterOutMax=[]  SumOutMin=[]  SumOutMax=[]  SumI1OutMin=[]  SumI1OutMax=[]  SumI2OutMin=[]  SumI2OutMax=[]  SumI3OutMin=[]  SumI3OutMax=[]  SumDOutMin=[]  SumDOutMax=[]  SaturationOutMin=[]  SaturationOutMax=[]  IntegratorContinuousStateAttributes=''  IntegratorStateMustResolveToSignalObject=off  IntegratorRTWStateStorageClass=Auto  FilterContinuousStateAttributes=''  FilterStateMustResolveToSignalObject=off  FilterRTWStateStorageClass=Auto  DifferentiatorICPrevScaledInput=0  DifferentiatorOutMin=[]  DifferentiatorOutMax=[]  InitialConditionSetting=State (most efficient)  FilterDiffOutCoefMin=[]  FilterDiffOutCoefMax=[]  SumDenOutMin=[]  SumDenOutMax=[]  SumNumOutMin=[]  SumNumOutMax=[]  ReciprocalOutMin=[]  ReciprocalOutMax=[]  DivideOutMin=[]  DivideOutMax=[]  TunerSelectOption=Transfer Function Based (PID Tuner App)
  PLL : powerlib_meascontrol/PLL/PLL  Fmin=45  Par_Init=[0, 60]  ParK=[180, 3200, 1]  TcD=1e-4  MaxRateChangeFreq=12  FilterCutOffFreq=25  Ts=0  AGC=on
      settings: SourceProductName=Simscape Power Systems  SourceProductBaseCode=PS
  PWM Generator (2-Level) : powerlib_meascontrol/Pulse & Signal Generators/PWM Generator (2-Level)  ModulatorType=Single-phase full-bridge (4 pulses)  ModulatorMode=Unsynchronized  Fc=10000  Pc=90  nF=27  MinMax="[ -1  1 ]"  SamplingTechnique=Natural  ModulatingSignals=off  m=0.8  Freq=60  Phase=0  Ts=0  ShowCarrierOutport=off
      settings: SourceProductName=Simscape Power Systems
  Product1 : Product  RndMeth=Zero
  Saturation1 : Saturate  UpperLimit=1  LowerLimit=-1
  Saturation3 : Saturate  UpperLimit=50  LowerLimit=-50
  Terminator : Terminator
  Transfer Fcn1 : TransferFcn  Denominator=[1e-4 1]
  Transfer Fcn2 : TransferFcn  Denominator=[1e-4 1]
  Transfer Fcn3 : TransferFcn  Denominator=[1e-4 1]
  Trigonometric Function : Trigonometry
  Pulse : Outport  OutputWhenDisabled=reset  InitialOutput=[0 0 0 0]
  wires:
  PWM Generator (2-Level)/1 -> Pulse/1
  370/1 -> Add1/2  "Vref"
  Add/1 -> PWM Generator (2-Level)/1  "duty_to_-1_1"
  Gain/1 -> Add/1
  Constant/1 -> Add/2
  V_Dc/1 -> Add1/1
  Add1/1 -> Transfer Fcn1/1  "err"
  I_Sys_Secondary/1 -> Add2/1
  Add2/1 -> Transfer Fcn2/1  "err"
  PID Controller1/1 -> Saturation1/1
  Transfer Fcn1/1 -> PID Controller/1  "Err_filter"
  Transfer Fcn2/1 -> PID Controller1/1  "err_filter"
  PID Controller/1 -> Saturation3/1  "Iref"
  Product1/1 -> Transfer Fcn3/1
  Saturation1/1 -> Gain/1
  Divide1/1 -> PLL/1  "V_Sys_Secondary"
  PLL/2 -> Trigonometric Function/1  "wt"
  Constant4/1 -> Divide1/2
  V_Sys_Secondary/1 -> Divide1/1
  Transfer Fcn3/1 -> Add2/2
  Saturation3/1 -> Product1/1
  Trigonometric Function/1 -> Product1/2
  PLL/1 -> Terminator/1  "Freq"

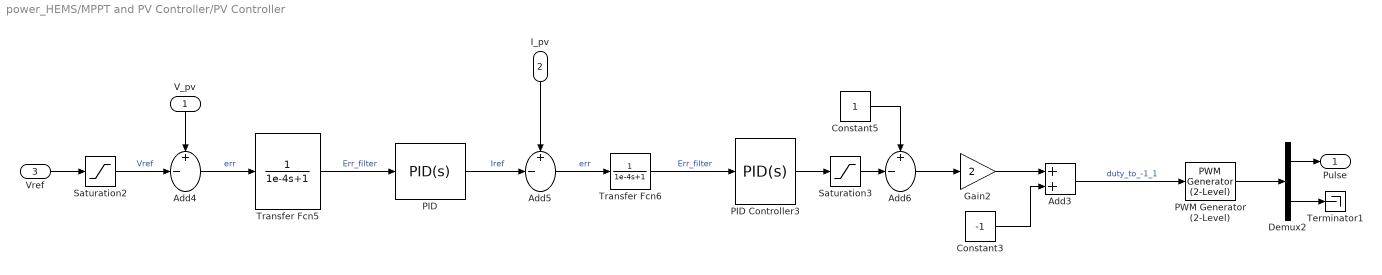
== system power_HEMS/MPPT and PV Controller/PV Controller ==
  V_pv : Inport
  I_pv : Inport  Port=2
  Vref : Inport  Port=3
  Add3 : Sum
  Add4 : Sum  Inputs=+-|
  Add5 : Sum  Inputs=+-|
  Add6 : Sum  Inputs=+-|
  Constant3 : Constant  Value=-1
  Constant5 : Constant
  Demux2 : Demux  Outputs=2
  Gain2 : Gain  Gain=2
  PID : simulink/Continuous/PID Controller  Controller=PID  TimeDomain=Continuous-time  SampleTime=-1  IntegratorMethod=Forward Euler  FilterMethod=Forward Euler  Form=Parallel  UseFilter=on  ControllerParametersSource=internal  P=Kp_V  I=Ki_V  D=0  N=100  InitialConditionSource=internal  InitialConditionForIntegrator=0  InitialConditionForFilter=0  ExternalReset=none  LimitOutput=off  UpperSaturationLimit=inf  LowerSaturationLimit=-inf  LinearizeAsGain=off  AntiWindupMode=none  Kb=1  TrackingMode=off  Kt=1  PParamMin=[]  PParamMax=[]  IParamMin=[]  IParamMax=[]  DParamMin=[]  DParamMax=[]  NParamMin=[]  NParamMax=[]  KbParamMin=[]  KbParamMax=[]  KtParamMin=[]  KtParamMax=[]  POutMin=[]  POutMax=[]  IOutMin=[]  IOutMax=[]  DOutMin=[]  DOutMax=[]  NOutMin=[]  NOutMax=[]  KbOutMin=[]  KbOutMax=[]  KtOutMin=[]  KtOutMax=[]  IntegratorOutMin=[]  IntegratorOutMax=[]  FilterOutMin=[]  FilterOutMax=[]  SumOutMin=[]  SumOutMax=[]  SumI1OutMin=[]  SumI1OutMax=[]  SumI2OutMin=[]  SumI2OutMax=[]  SumI3OutMin=[]  SumI3OutMax=[]  SumDOutMin=[]  SumDOutMax=[]  SaturationOutMin=[]  SaturationOutMax=[]  IntegratorContinuousStateAttributes=''  IntegratorStateMustResolveToSignalObject=off  IntegratorRTWStateStorageClass=Auto  FilterContinuousStateAttributes=''  FilterStateMustResolveToSignalObject=off  FilterRTWStateStorageClass=Auto  DifferentiatorICPrevScaledInput=0  DifferentiatorOutMin=[]  DifferentiatorOutMax=[]  InitialConditionSetting=State (most efficient)  FilterDiffOutCoefMin=[]  FilterDiffOutCoefMax=[]  SumDenOutMin=[]  SumDenOutMax=[]  SumNumOutMin=[]  SumNumOutMax=[]  ReciprocalOutMin=[]  ReciprocalOutMax=[]  DivideOutMin=[]  DivideOutMax=[]  TunerSelectOption=Transfer Function Based (PID Tuner App)
  PID Controller3 : simulink/Continuous/PID Controller  Controller=PID  TimeDomain=Continuous-time  SampleTime=-1  IntegratorMethod=Forward Euler  FilterMethod=Forward Euler  Form=Parallel  UseFilter=on  ControllerParametersSource=internal  P=Kp_I  I=Ki_I  D=0  N=100  InitialConditionSource=internal  InitialConditionForIntegrator=0  InitialConditionForFilter=0  ExternalReset=none  LimitOutput=off  UpperSaturationLimit=inf  LowerSaturationLimit=-inf  LinearizeAsGain=off  AntiWindupMode=none  Kb=1  TrackingMode=off  Kt=1  PParamMin=[]  PParamMax=[]  IParamMin=[]  IParamMax=[]  DParamMin=[]  DParamMax=[]  NParamMin=[]  NParamMax=[]  KbParamMin=[]  KbParamMax=[]  KtParamMin=[]  KtParamMax=[]  POutMin=[]  POutMax=[]  IOutMin=[]  IOutMax=[]  DOutMin=[]  DOutMax=[]  NOutMin=[]  NOutMax=[]  KbOutMin=[]  KbOutMax=[]  KtOutMin=[]  KtOutMax=[]  IntegratorOutMin=[]  IntegratorOutMax=[]  FilterOutMin=[]  FilterOutMax=[]  SumOutMin=[]  SumOutMax=[]  SumI1OutMin=[]  SumI1OutMax=[]  SumI2OutMin=[]  SumI2OutMax=[]  SumI3OutMin=[]  SumI3OutMax=[]  SumDOutMin=[]  SumDOutMax=[]  SaturationOutMin=[]  SaturationOutMax=[]  IntegratorContinuousStateAttributes=''  IntegratorStateMustResolveToSignalObject=off  IntegratorRTWStateStorageClass=Auto  FilterContinuousStateAttributes=''  FilterStateMustResolveToSignalObject=off  FilterRTWStateStorageClass=Auto  DifferentiatorICPrevScaledInput=0  DifferentiatorOutMin=[]  DifferentiatorOutMax=[]  InitialConditionSetting=State (most efficient)  FilterDiffOutCoefMin=[]  FilterDiffOutCoefMax=[]  SumDenOutMin=[]  SumDenOutMax=[]  SumNumOutMin=[]  SumNumOutMax=[]  ReciprocalOutMin=[]  ReciprocalOutMax=[]  DivideOutMin=[]  DivideOutMax=[]  TunerSelectOption=Transfer Function Based (PID Tuner App)
  PWM Generator (2-Level) : powerlib_meascontrol/Pulse & Signal Generators/PWM Generator (2-Level)  ModulatorType=Single-phase full-bridge (4 pulses)  ModulatorMode=Unsynchronized  Fc=10000  Pc=90  nF=27  MinMax="[ -1  1 ]"  SamplingTechnique=Natural  ModulatingSignals=off  m=0.8  Freq=60  Phase=0  Ts=0  ShowCarrierOutport=off
      settings: SourceProductName=Simscape Power Systems
  Saturation2 : Saturate  UpperLimit=280  LowerLimit=0
  Saturation3 : Saturate  UpperLimit=1  LowerLimit=0
  Terminator1 : Terminator
  Transfer Fcn5 : TransferFcn  Denominator=[1e-4 1]
  Transfer Fcn6 : TransferFcn  Denominator=[1e-4 1]
  Pulse : Outport
  wires:
  PWM Generator (2-Level)/1 -> Demux2/1
  Vref/1 -> Saturation2/1
  I_pv/1 -> Add5/1
  Add3/1 -> PWM Generator (2-Level)/1  "duty_to_-1_1"
  Gain2/1 -> Add3/1
  Constant3/1 -> Add3/2
  Demux2/2 -> Terminator1/1
  Saturation2/1 -> Add4/2  "Vref"
  Add4/1 -> Transfer Fcn5/1  "err"
  PID/1 -> Add5/2  "Iref"
  Add5/1 -> Transfer Fcn6/1  "err"
  PID Controller3/1 -> Saturation3/1
  Saturation3/1 -> Add6/2
  Constant5/1 -> Add6/1
  Add6/1 -> Gain2/1
  Transfer Fcn5/1 -> PID/1  "Err_filter"
  Transfer Fcn6/1 -> PID Controller3/1  "Err_filter"
  V_pv/1 -> Add4/1
  Demux2/1 -> Pulse/1

== system power_HEMS/MPPT and PV Controller/PWM Controller 2 ==
  Vdc : Inport
  Enable : EnablePort  StatesWhenEnabling=reset
  Add : Sum
  Constant : Constant  Value=200*sqrt(2)
  Constant1 : Constant  Value=1e-6
  Divide : Product  Inputs=*/
  PWM Generator (2-Level) : powerlib_meascontrol/Pulse & Signal Generators/PWM Generator (2-Level)  ModulatorType=Single-phase full-bridge (4 pulses)  ModulatorMode=Unsynchronized  Fc=10000  Pc=90  nF=27  MinMax="[ -1  1 ]"  SamplingTechnique=Natural  ModulatingSignals=off  m=0.8  Freq=60  Phase=0  Ts=0  ShowCarrierOutport=off
      settings: SourceProductName=Simscape Power Systems
  Product2 : Product  SampleTime=5e-6  RndMeth=Zero
  Uref Generation (60Hz) : Sin  Frequency=2*pi*60  SampleTime=5e-6
  Pulse : Outport  OutputWhenDisabled=reset  InitialOutput=[0 0 0 0]
  wires:
  PWM Generator (2-Level)/1 -> Pulse/1
  Product2/1 -> PWM Generator (2-Level)/1
  Uref Generation (60Hz)/1 -> Product2/2
  Divide/1 -> Product2/1
  Vdc/1 -> Add/1
  Constant/1 -> Divide/1
  Constant1/1 -> Add/2
  Add/1 -> Divide/2

== system power_HEMS/Scenario/Load switching ==
  Demux : Demux  Tag=STV Demux  Outputs=2
  FromWs : FromWorkspace  Tag=STV FromWs  VariableName=tuvar  SampleTime=0
      SigBuilderData=|
      | common.afterFinalStr = 'Extrapolate'
      | common.sampleTime = 0
      | dataSet.timeRange = [0 10]
      | dataSet.name = 'Group 1'
      | sbobj.Groups.Name = 'Group 1'
      | sbobj.Groups.Signals(1).Name = 'Load 1'
      | sbobj.Groups.Signals(1).XData = [0 0.5 0.5 1.5 1.5 2.5 2.5 3.5 3.5 4 10]
      | sbobj.Groups.Signals(1).YData = [0 0 1 1 0 0 1 1 0 0 0]
      | sbobj.Groups.Signals(2).Name = 'Load 2'
      | sbobj.Groups.Signals(2).XData = [0 1 1 1.5 1.5 3 3 3.5 3.5 10]
      | sbobj.Groups.Signals(2).YData = [0 0 1 1 0 0 1 1 0 0]
  Load 1 : Outport  Tag=STV Outport
  Load 2 : Outport  Tag=STV Outport  Port=2
  wires:
  Demux/1 -> Load 1/1
  FromWs/1 -> Demux/1
  Demux/2 -> Load 2/1

== system power_HEMS/Scenario/Power source ==
  Demux : Demux  Tag=STV Demux  Outputs=1
  FromWs : FromWorkspace  Tag=STV FromWs  VariableName=tuvar  SampleTime=0
      SigBuilderData=|
      | common.afterFinalStr = 'Extrapolate'
      | common.sampleTime = 0
      | dataSet.timeRange = [0 10]
      | dataSet.name = 'Group 1'
      | sbobj.Groups.Name = 'Group 1'
      | sbobj.Groups.Signals.Name = 'Signal 2'
      | sbobj.Groups.Signals.XData = [0 2 2 4 4 10]
      | sbobj.Groups.Signals.YData = [1 1 0 0 1 1]
  Signal 2 : Outport  Tag=STV Outport
  wires:
  Demux/1 -> Signal 2/1
  FromWs/1 -> Demux/1

== stateflow chart power_HEMS/MPPT and PV Controller/MPPT Controller ==
  settings: updateMethod=DISCRETE  sampleTime=5e-3
  state MPPT/
    (default) -> (junction 64)
    MPPT -> (junction 64)
    (junction 64) -> (junction 62) : {P_pv = I_pv*V_pv;}
    (junction 62) -> (junction 54) [order 2]
    (junction 62) -> (junction 61) [order 1] : [Last_P_pv >= P_pv]
        | {Vref = Vref - dV;}
    (junction 54) -> (junction 59) : [Last_P_pv < P_pv]
        | {Vref = Vref + dV;}
    (junction 59) -> (junction 61)
    (junction 61) -> (junction 52) : {Last_P_pv = P_pv;}
  (default) -> MPPT
  data: V_pv input; I_pv input; Last_P_pv local double; P_pv local double; Vref output double =200; dV parameter double
